simulink model "P1"  (R2023b)
settings: Solver=VariableStepAuto  StartTime=0.0  StopTime=10.0  RelTol=1e-3
libraries: SignalEditorBlockLib x1
settings Model: Creator=Usuario_UMA  LastModifiedBy=Usuario_UMA

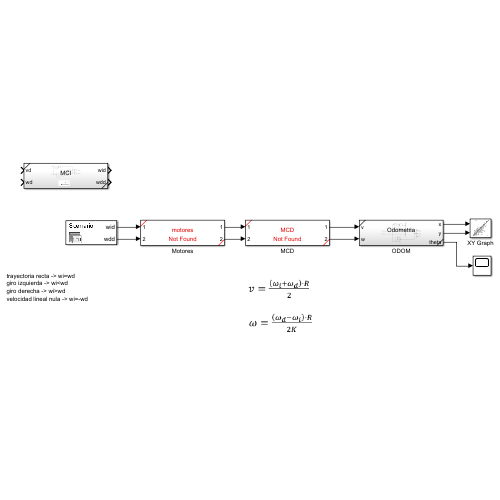
[thumbnail: Simulink's stored preview of the top-level diagram]
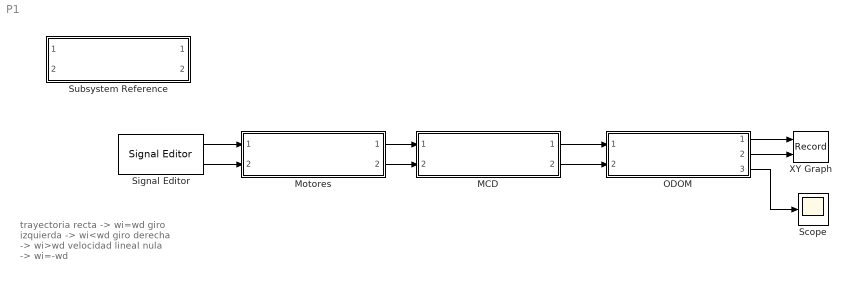
== system P1 ==
  note: trayectoria recta -> wi=wd
      | giro izquierda -> wi<wd
      | giro derecha -> wi>wd
      | velocidad lineal nula -> wi=-wd
  MCD : Subsystem  ReferencedSubsystem=MCD
  Motores : Subsystem  ReferencedSubsystem=motores
  ODOM : Subsystem  ReferencedSubsystem=Odometria
  Scope : Scope
  Signal Editor : SignalEditorBlockLib/Signal Editor  FileName=giro_izquierda.mat  ActiveScenario=Scenario  ActiveSignal=wid  IsBus=off  OutputBusObjectStr=Bus: BusObject  SampleTime=0  Interpolate=off  ZeroCross=off  OutputAfterFinalValue=Setting to zero  Unit=inherit  PreserveSignalName=on  ApplySigPropsToAllScenarios=on  ApplySigPropsToAllSignals=off
  Subsystem Reference : Subsystem  ReferencedSubsystem=MCI
  XY Graph : Record  FileSettingsInternal="{\"entries\":[{\"content\":{\"excelSettings\":{\"content\":{},\"type\":\"Streamout.ExcelSettings\"}},\"type\":\"Streamout.FileSettingStorage\",\"uuid\":\"\"}],\"packageUris\":[\"http:\\/\\/schema.mathworks.com\\/mf0\\/streamout_blocks\\/R2020a\"],\"version\":\"1.0\"}"  Layout=[1 1]  SignalsInternal="{\"entries\":[{\"content\":{\"signals\":[{\"content\":{\"blockPath\":[],\"dimensions\":[1],\"domain\":\"\",\"lineColor\":\"#a2142f\",\"plots\":[1],\"port\":1,\"signalID\":17,\"signalName\":\"ODOM:1\"},\"type\":\"RecordBlkView.Signal\",\"uuid\":\"\"},{\"content\":{\"blockPath\":[],\"dimensions\":[1],\"domain\":\"\",\"lineColor\":\"#139fff\",\"plots\":[1],\"port\":2,\"signalID\":20,\"signalName\":\"ODOM:2\"},\"type\":\"RecordBlkView.Signal\",\"uuid\":\"\"}]},\"type\":\"RecordBlkView.InputSignals\",\"uuid\":\"\"}],\"packageUris\":[\"http:\\/\\/schema.mathworks.com\\/mf0\\/streamout_blocks\\/R2020a\"],\"version\":\"1.0\"}"  VisualizationBindings="{\"xyplotplugin\":{\"info\":[{\"series\":[{\"bindingParametersList\":[{\"parameter\":\"X-Axis\",\"signalID\":17,\"signalName\":\"ODOM:1\"},{\"parameter\":\"Y-Axis\",\"signalID\":20,\"signalName\":\"ODOM:2\"}],\"seriesID\":58680}],\"subplotID\":1}]}}"  CompatibilityTag=XY
  wires:
  MCD/1 -> ODOM/1
  MCD/2 -> ODOM/2
  ODOM/1 -> XY Graph/1
  ODOM/2 -> XY Graph/2
  Motores/1 -> MCD/1
  Motores/2 -> MCD/2
  Signal Editor/1 -> Motores/1
  Signal Editor/2 -> Motores/2
  ODOM/3 -> Scope/1
